simulink model "Problem2"  (R2020b)
settings: Solver=VariableStepAuto  StartTime=0.0  StopTime=10.0  RelTol=1e-3
undefined symbols (not defined in the file): b, k1, k2, m1, m2
settings Model: Creator=Dell  LastModifiedBy=Dell

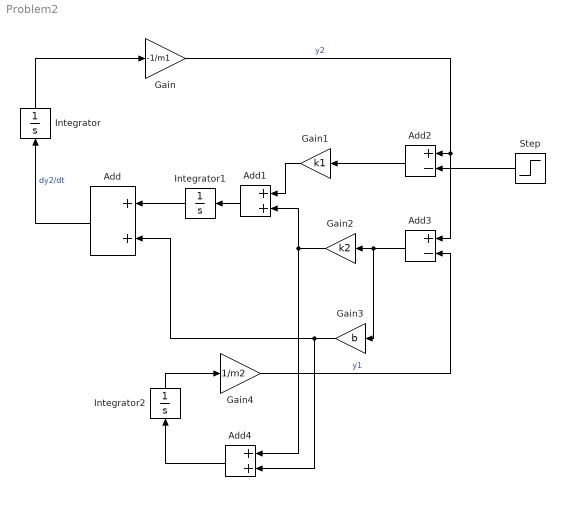
== system Problem2 ==
  Add : Sum
  Add1 : Sum
  Add2 : Sum  Inputs=+-
  Add3 : Sum  Inputs=+-
  Add4 : Sum
  Gain : Gain  Gain=-1/m1
  Gain1 : Gain  Gain=k1
  Gain2 : Gain  Gain=k2
  Gain3 : Gain  Gain=b
  Gain4 : Gain  Gain=1/m2
  Integrator : Integrator
  Integrator1 : Integrator
  Integrator2 : Integrator
  Step : Step  SampleTime=0
  wires:
  Gain1/1 -> Add1/1
  Gain2/1 -> Add4/1, Add1/2
  Add/1 -> Integrator/1  "dy2/dt"
  Integrator/1 -> Gain/1
  Step/1 -> Add2/2
  Gain/1 -> Add3/1, Add2/1  "y2"
  Add2/1 -> Gain1/1
  Add3/1 -> Gain3/1, Gain2/1
  Integrator1/1 -> Add/1
  Add1/1 -> Integrator1/1
  Gain3/1 -> Add4/2, Add/2
  Add4/1 -> Integrator2/1
  Integrator2/1 -> Gain4/1
  Gain4/1 -> Add3/2  "y1"
